simulink model "turbine_th"  (R2018b)
settings: Solver=VariableStepAuto  StartTime=0.0  StopTime=0  RelTol=1e-3
values from neighbouring files (symbols this model uses):
  angVecBdy = [0 0 -1]    [turbine_ts.m]
  velVecBdy = [0 0 0]    [turbine_ts.m]
  vWindBdy = [0 0 0]    [turbine_ts.m]
libraries: turbine_ul x1
settings Model: Creator=mcobb  LastModifiedBy=mcobb

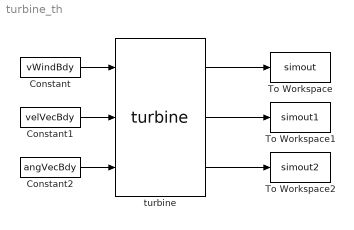
== system turbine_th ==
  Constant : Constant  Value=vWindBdy
  Constant1 : Constant  Value=velVecBdy
  Constant2 : Constant  Value=angVecBdy
  To Workspace : ToWorkspace  VariableName=simout  SaveFormat=Timeseries  SampleTime=-1
  To Workspace1 : ToWorkspace  VariableName=simout1  SaveFormat=Timeseries  SampleTime=-1
  To Workspace2 : ToWorkspace  VariableName=simout2  SaveFormat=Timeseries  SampleTime=-1
  turbine : turbine_ul/turbine  diam=d  Cp=Cp  Cd=Cd  rho=rho  rTurb=turbPosVec
  wires:
  Constant/1 -> turbine/1
  turbine/1 -> To Workspace/1
  turbine/2 -> To Workspace1/1
  turbine/3 -> To Workspace2/1
  Constant1/1 -> turbine/2
  Constant2/1 -> turbine/3
